simulink model "Exp_07_01_02"  (R2012b)
settings: Solver=ode45  StartTime=0.0  StopTime=10.0  MaxStep=0.01  RelTol=1e-3
settings Model: Creator=Abraham Xiao  LastModifiedBy=Abraham Xiao
settings RTWCC: GenerateReport=on  LaunchReport=on
settings CodeAppCC: ForceParamTrailComments=on  MATLABSourceComments=on

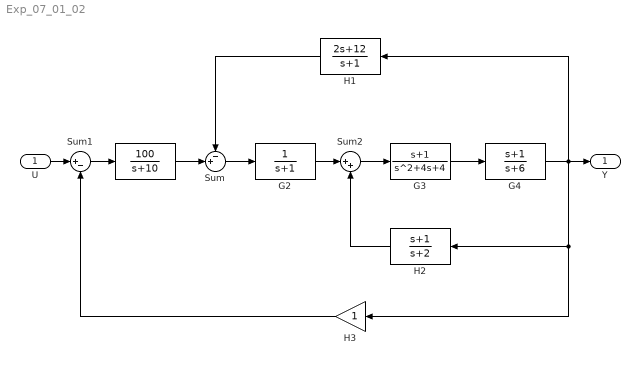
== system Exp_07_01_02 ==
  U : Inport
  " " : TransferFcn  Numerator=[100]  Denominator=[1 10]
  " H1" : TransferFcn  Numerator=[2 12]  Denominator=[1 1]
  "G2 " : TransferFcn  Denominator=[1 1]
  G3 : TransferFcn  Numerator=[1, 1]  Denominator=[1, 4, 4]
  G4 : TransferFcn  Numerator=[1 1]  Denominator=[1 6]
  H2 : TransferFcn  Numerator=[1 1]  Denominator=[1 2]
  H3 : Gain
  Sum : Sum  Inputs=-+|
  Sum1 : Sum  Inputs=|+-
  Sum2 : Sum  Inputs=|++
  Y : Outport
  wires:
  U/1 -> Sum1/1
  Sum1/1 -> " "/1
  " "/1 -> Sum/2
  Sum/1 -> "G2 "/1
  "G2 "/1 -> Sum2/1
  Sum2/1 -> G3/1
  G3/1 -> G4/1
  G4/1 -> " H1"/1, H3/1, H2/1, Y/1
  H2/1 -> Sum2/2
  H3/1 -> Sum1/2
  " H1"/1 -> Sum/1
